simulink model "prova"  (R2020a)
settings: Solver=ode45  StartTime=0.0  StopTime=0.7  RelTol=1e-3
values from neighbouring files (symbols this model uses):
  b_ck = 0.03    [Parameters.m]
  b_cv = 0.03    [Parameters.m]
  Jc = 0.01    [Parameters.m]
  Jeq = 0.5*(Je/(tauf)+M*Rw^2+4*Jw)    (= 39.7521)    [Parameters.m]
  k = 0.098    [Parameters.m]
  T_eq = -200    [Parameters.m]
  T_l = 0    [Parameters.m]
  v = (control.F(1))\(-control.U(:,:,1)*x_0 - control.K(1))    [Parameters.m]
  x_0 = [90;90;0]    [Parameters.m]
settings Model: Creator=andre  LastModifiedBy=andre

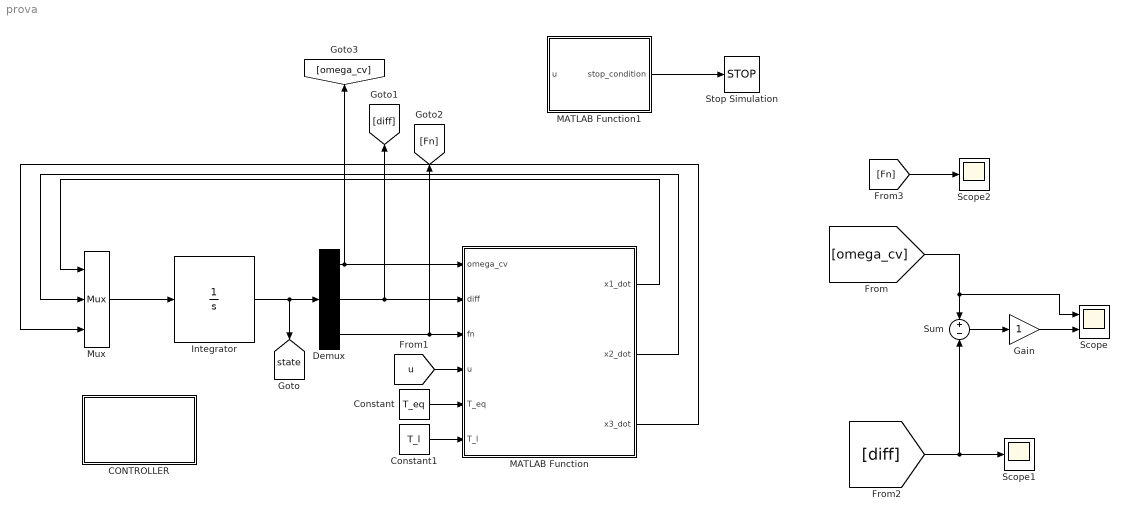
== system prova ==
  CONTROLLER : Subsystem
  Constant : Constant  Value=T_eq
  Constant1 : Constant  Value=T_l
  Demux : Demux  Outputs=3
  Gain : Gain
  Integrator : Integrator  InitialCondition=x_0
  MATLAB Function : MATLAB Function  TreatAsAtomicUnit=on
  MATLAB Function1 : MATLAB Function  TreatAsAtomicUnit=on
  Mux : Mux  Inputs=3
  Scope : Scope  NumInputPorts=2
  Scope1 : Scope
  Scope2 : Scope
  Stop Simulation : Stop
  Sum : Sum  Inputs=+-
  tag scope: state=global
  wires:
  Mux/1 -> Integrator/1
  Integrator/1 -> Demux/1, [state]
  MATLAB Function/1(x1_dot) -> Mux/1
  MATLAB Function/2(x2_dot) -> Mux/2
  MATLAB Function/3(x3_dot) -> Mux/3
  Demux/2 -> MATLAB Function/2(diff), [diff]
  Demux/3 -> [Fn], MATLAB Function/3(fn)
  MATLAB Function1/1(stop_condition) -> Stop Simulation/1
  Constant/1 -> MATLAB Function/5(T_eq)
  Constant1/1 -> MATLAB Function/6(T_l)
  [u] -> MATLAB Function/4(u)
  Demux/1 -> MATLAB Function/1(omega_cv), [omega_cv]
  [Fn] -> Scope2/1
  [diff] -> Sum/2, Scope1/1
  [omega_cv] -> Scope/1, Sum/1
  Sum/1 -> Gain/1
  Gain/1 -> Scope/2

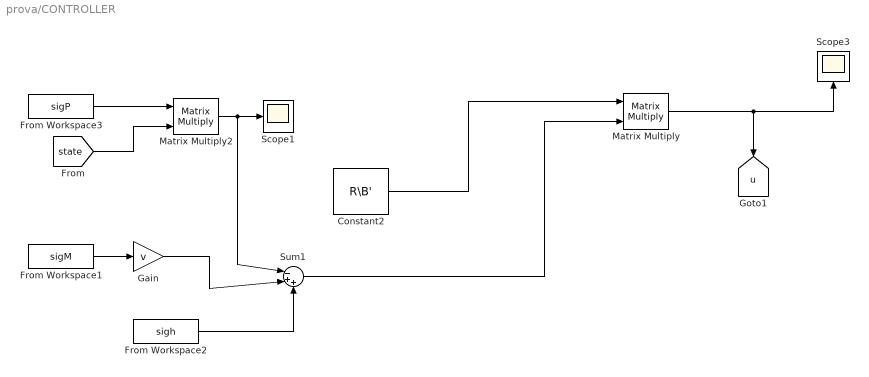
== system prova/CONTROLLER ==
  Constant2 : Constant  Value=R\B'  VectorParams1D=off
  From Workspace1 : FromWorkspace  VariableName=sigM
  From Workspace2 : FromWorkspace  VariableName=sigh
  From Workspace3 : FromWorkspace  VariableName=sigP
  Gain : Gain  Gain=v
  Matrix Multiply : Product  Multiplication=Matrix(*)
  Matrix Multiply2 : Product  Multiplication=Matrix(*)
  Scope1 : Scope
  Scope3 : Scope
  Sum1 : Sum  Inputs=|-++
  tag scope: u=global
  wires:
  Matrix Multiply2/1 -> Sum1/1, Scope1/1
  Matrix Multiply/1 -> [u], Scope3/1
  Gain/1 -> Sum1/2
  From Workspace2/1 -> Sum1/3
  From Workspace1/1 -> Gain/1
  Sum1/1 -> Matrix Multiply/2
  Constant2/1 -> Matrix Multiply/1
  From Workspace3/1 -> Matrix Multiply2/1
  [state] -> Matrix Multiply2/2

== matlab function prova/MATLAB Function1 ==
  data: u input; stop_condition output
function stop_condition = stop(u)
    threshold = 1e-2;
    stop_condition = 0;
    if u < threshold 
        stop_condition = 1;
    end
end

== matlab function prova/MATLAB Function ==
  data: omega_cv input; x1_dot output; diff input; fn input; u input; T_eq input; T_l input; x2_dot output; Jeq parameter; Jc parameter; b_cv parameter; b_ck parameter; k parameter; x3_dot output
function [x1_dot,x2_dot,x3_dot] = dynamics(omega_cv,diff,fn,...
    u,T_eq,T_l,Jeq,Jc,b_cv, b_ck, k)

    x1 = omega_cv;
    x2 = diff;
    x3 = fn;
    Jeq = 3;
    x1_dot = 1/Jeq*(-b_cv*x1 + T_eq - k*x3);
    x2_dot = (-b_cv/Jeq+b_ck/Jc)*x1 -(b_ck/Jc)*x2 -(k/Jeq+k/Jc)*x3+...
        T_eq/Jeq + T_l/Jc; 
    x3_dot = u;
    
end
